simulink subsystem "Controller"  (R2025a)
settings: Solver=VariableStepAuto  StartTime=0.0  StopTime=10.0  RelTol=1e-3
undefined symbols (not defined in the file): DiscIntNeverNeededParam
settings Model: Creator=kvasios  LastModifiedBy=kvasios

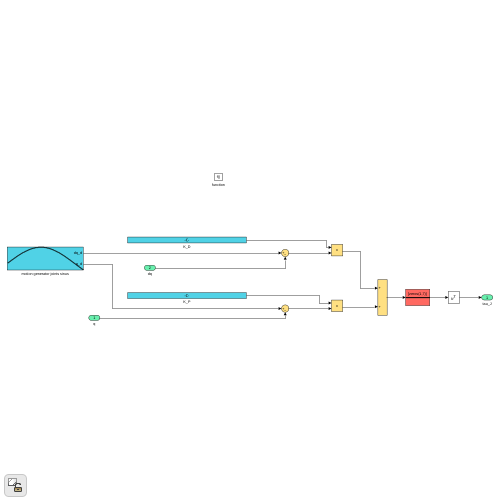
[thumbnail: Simulink's stored preview of the top-level diagram]
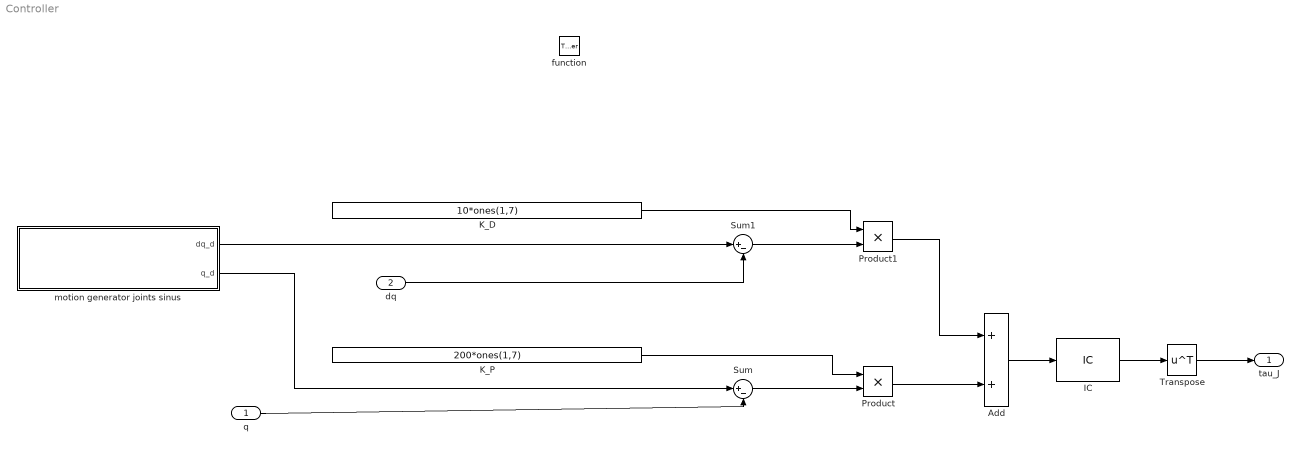
== system Controller ==
  q : Inport
  dq : Inport  Port=2
  function : TriggerPort  TriggerType=function-call  VariantControl=(inherit)
  Add : Sum
  IC : InitialCondition  Value=zeros(1,7)
  K_D : Constant  Value=10*ones(1,7)  VectorParams1D=off  SampleTime=-1
  K_P : Constant  Value=200*ones(1,7)  VectorParams1D=off  SampleTime=-1
  Product : Product
  Product1 : Product
  Sum : Sum  Inputs=|+-
  Sum1 : Sum  Inputs=|+-
  Transpose : Math  Operator=transpose
  motion generator joints sinus : Subsystem
      mask Display:
      | pos = get_param(gcb, 'Position');
      | width = pos(3) - pos(1);
      | x = [0:width];
      | y = sin(x/180*pi);
      | % Parameters 'm' and 'b' must be defined in 'Parameters & Dialog' pane.
      | plot(x,y );
      | 
      | port_label('output',1,'dq_d');
      | port_label('output',2,'q_d');
  tau_J : Outport  VectorParamsAs1DForOutWhenUnconnected=off
  wires:
  IC/1 -> Transpose/1
  Add/1 -> IC/1
  Sum1/1 -> Product1/2
  motion generator joints sinus/1(dq_d) -> Sum1/1
  Product1/1 -> Add/1
  Product/1 -> Add/2
  K_D/1 -> Product1/1
  K_P/1 -> Product/1
  Sum/1 -> Product/2
  Transpose/1 -> tau_J/1
  dq/1 -> Sum1/2
  motion generator joints sinus/2(q_d) -> Sum/1
  q/1 -> Sum/2

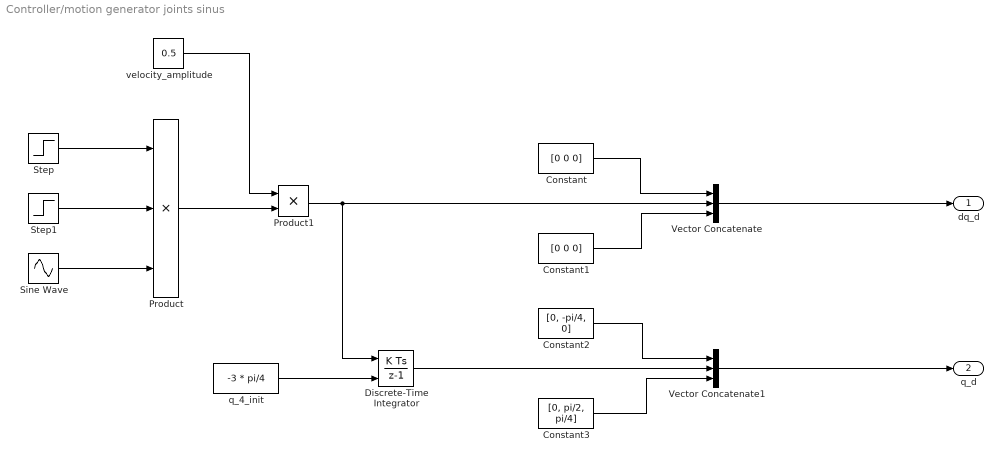
== system Controller/motion generator joints sinus ==
  Constant : Constant  Value=[0 0 0]  VectorParams1D=off
  Constant1 : Constant  Value=[0 0 0]  VectorParams1D=off
  Constant2 : Constant  Value=[0, -pi/4, 0]  VectorParams1D=off
  Constant3 : Constant  Value=[0, pi/2, pi/4]  VectorParams1D=off
  Discrete-Time Integrator : DiscreteIntegrator  InitialConditionSource=external  SampleTime=-1  ICPrevOutput=DiscIntNeverNeededParam  ICPrevScaledInput=DiscIntNeverNeededParam
  Product : Product  Inputs=3
  Product1 : Product
  Sine Wave : Sin  Frequency=pi  Phase=pi
  Step : Step
  Step1 : Step  Time=7  Before=1  After=0
  Vector Concatenate : Concatenate  NumInputs=3
  Vector Concatenate1 : Concatenate  NumInputs=3
  q_4_init : Constant  Value=-3 * pi/4  VectorParams1D=off
  velocity_amplitude : Constant  Value=0.5  VectorParams1D=off
  dq_d : Outport  VectorParamsAs1DForOutWhenUnconnected=off
  q_d : Outport  Port=2  VectorParamsAs1DForOutWhenUnconnected=off
  wires:
  Step1/1 -> Product/2
  q_4_init/1 -> Discrete-Time Integrator/2
  Vector Concatenate1/1 -> q_d/1
  Discrete-Time Integrator/1 -> Vector Concatenate1/2
  Constant2/1 -> Vector Concatenate1/1
  Constant3/1 -> Vector Concatenate1/3
  Vector Concatenate/1 -> dq_d/1
  Product1/1 -> Vector Concatenate/2, Discrete-Time Integrator/1
  velocity_amplitude/1 -> Product1/1
  Step/1 -> Product/1
  Sine Wave/1 -> Product/3
  Product/1 -> Product1/2
  Constant/1 -> Vector Concatenate/1
  Constant1/1 -> Vector Concatenate/3
